simulink model "Simscape_CAD_SLIP"  (R2022a)
settings: Solver=VariableStepAuto  StartTime=0.0  StopTime=4  FixedStep=1E-6  MaxStep=1E-5  RelTol=1E-9
undefined symbols (not defined in the file or in its folder): arm_l, arm_r, arm_spacing, base_h, base_r, desired_speed, equilibrium_length, height_plane, hip_fuzz, initHip, initKnee, k_landing_angle, k_slip, knee_fuzz, lower_leg_length, max_torque, plane_x, plane_y, plane_z, upper_leg_length, X, Y, Z
libraries: sm_lib x46, nesl_utility x14, slpidlib x4, simulink x1
(part 3 of 3)

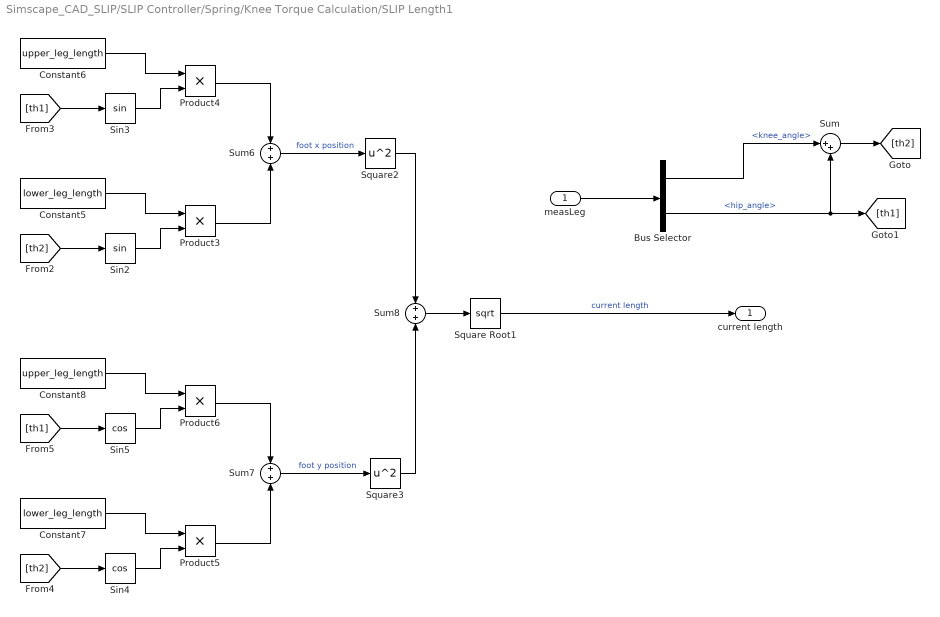
== system Simscape_CAD_SLIP/SLIP Controller/Spring/Knee Torque Calculation/SLIP Length1 ==
  measLeg : Inport
  Bus Selector : BusSelector  OutputSignals=knee_angle,hip_angle
  Constant5 : Constant  Value=lower_leg_length
  Constant6 : Constant  Value=upper_leg_length
  Constant7 : Constant  Value=lower_leg_length
  Constant8 : Constant  Value=upper_leg_length
  Product{3..6} (4 alike) : Product
  Sin2 : Trigonometry
  Sin3 : Trigonometry
  Sin4 : Trigonometry  Operator=cos
  Sin5 : Trigonometry  Operator=cos
  Square Root1 : Sqrt
  Square2 : Math  Operator=square
  Square3 : Math  Operator=square
  Sum : Sum  Inputs=|++
  Sum6 : Sum  Inputs=+|+
  Sum7 : Sum  Inputs=+|+
  Sum8 : Sum  Inputs=+|+
  current length : Outport
  wires:
  Square2/1 -> Sum8/1
  Sum7/1 -> Square3/1  "foot y position"
  [th2] -> Sin2/1
  Square3/1 -> Sum8/2
  Sin4/1 -> Product5/2
  Constant5/1 -> Product3/1
  Constant7/1 -> Product5/1
  Product6/1 -> Sum7/1
  Product3/1 -> Sum6/2
  [th2] -> Sin4/1
  Product5/1 -> Sum7/2
  [th1] -> Sin5/1
  Sin3/1 -> Product4/2
  Constant8/1 -> Product6/1
  Sin5/1 -> Product6/2
  Sin2/1 -> Product3/2
  Sum6/1 -> Square2/1  "foot x position"
  Constant6/1 -> Product4/1
  Product4/1 -> Sum6/1
  Sum8/1 -> Square Root1/1
  [th1] -> Sin3/1
  Square Root1/1 -> current length/1  "current length"
  Bus Selector/1 -> Sum/1  "<knee_angle>"
  Bus Selector/2 -> Sum/2, [th1]  "<hip_angle>"
  measLeg/1 -> Bus Selector/1
  Sum/1 -> [th2]

== stateflow chart Simscape_CAD_SLIP/SLIP Controller ==
  state Flight
  state Unload
  state Load
  state Idle
  state Spring
  Unload -> Flight : [after(5,msec)]{contactTime = simTime(end)-landingTime,n=n+1,hasHopped = 1}
  Flight -> Load : [Simscape_Transitions>1]{SLIP_impact_angle = atan(foot_x_flight(end)/foot_y_flight(end)),landingTime=simTime(end)}
  (default) -> Idle : {n=0,loopchecks = zeros(1,2), contactTime = 0,hasHopped = 0,landingTime = 0}
  Load -> Idle [order 2] : [run == 0]
  Idle -> Load : [run == 1]
  Spring -> Unload : [Simscape_Transitions<1]
  Load -> Spring [order 1] : [after(5,msec)]
  data: sf_internal_action_state_placeholder_data local double size=1 =0; sf_internal_action_state_placeholder_data local double size=1 =0; sf_internal_action_state_placeholder_data local double size=1 =0; sf_internal_action_state_placeholder_data local double size=1 =0; sf_internal_action_state_placeholder_data local double size=1 =0; InputL output; measLeg input; measBody input; contactTime data_store_memory; Simscape_Transitions data_store_memory; Machine_State output; n output; loopchecks output; foot_x_flight data_store_memory; foot_y_flight data_store_memory; SLIP_impact_angle data_store_memory; simTime data_store_memory; landingTime local; hasHopped data_store_memory; run data_store_memory
